simulink model "beta2"  (R2018b)
settings: Solver=FixedStepDiscrete  StartTime=0.0  StopTime=inf  FixedStep=.001  RelTol=1e-3
StartFcn:
  | system('iRobotisManipulator.exe RobotisManipulator_ctr &')
libraries: LibrarySimulinkSAS x4, aerolibanimutils x1
settings Model: SimulationMode=accelerator  Creator=dds  LastModifiedBy=dds
settings OptimizationCC: LifeSpan=inf
settings DebuggingCC: LibraryContextMissingDiagnostic=none  SFExecutionAtInitializationDiag=none
settings SFSimCC: SimUseLocalCustomCode=off
settings RTWCC: RTWUseLocalCustomCode=off
settings CodeAppCC: StateflowObjectComments=on

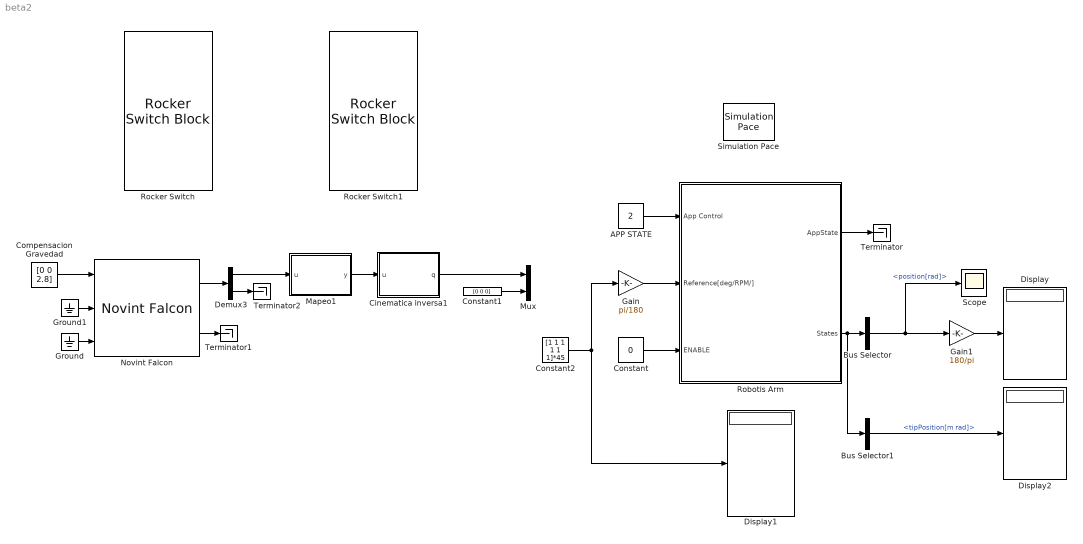
== system beta2 ==
  APP STATE : Constant  Value=2
  Bus Selector : BusSelector  OutputSignals=position[rad]
  Bus Selector1 : BusSelector  OutputSignals=tipPosition[m rad]
  Cinematica inversa1 : MATLAB Function  TreatAsAtomicUnit=on
  Compensacion Gravedad : Constant  Value=[0 0 2.8]  SampleTime=-1
  Constant : Constant  Value=0
  Constant1 : Constant  Value=[0 0 0]
  Constant2 : Constant  Value=[1 1 1 1 1 1]*45
  Demux3 : Demux  Outputs=2
  Display : Display
  Display1 : Display
  Display2 : Display
  Gain : Gain  Gain=pi/180
  Gain1 : Gain  Gain=180/pi
  Ground : Ground
  Ground1 : Ground
  Mapeo1 : MATLAB Function  TreatAsAtomicUnit=on
  Mux : Mux  Inputs=2
  Novint Falcon : LibrarySimulinkSAS/Novint Falcon  dev=1
      settings: SourceProductName=Library SAS
  Robotis Arm : Subsystem  mask{port='COM3', baud='3000000', tloop=10000, ctrType='CTR_POSITION'}
      mask prompts: baud "Baudrate"; tloop "Sample Time [us]"; ctrType "Control Type"
      mask Display:
      | image('robotis.jpg')
      | color('red');
      | port_label('output', 1, 'App ctr State' )
      | port_label('output', 2, 'Robot States' )
      | color('blue');
      | port_label('input', 1, 'App Control')
      | port_label('input', 2, 'Reference [rad]')
      | port_label('input', 3, 'Enable')
      | port_label('input', 4, 'Planes Restriction')
  Rocker Switch : RockerSwitchBlock  WebBlockId=161
      settings: Values={{'CLOSE', 'START'}, [5 2]}
  Rocker Switch1 : RockerSwitchBlock  WebBlockId=162
      settings: Values={{'Motors OFF', 'Motors ON'}, [0 1]}
  Scope : Scope
  Simulation Pace : aerolibanimutils/Simulation Pace  SimulationPace=1  SleepMode=MATLAB Thread  OutputPaceError=off  SampleTime=-1
  Terminator : Terminator
  Terminator1 : Terminator
  Terminator2 : Terminator
  wires:
  APP STATE/1 -> Robotis Arm/1(App Control)
  Constant/1 -> Robotis Arm/3(ENABLE)
  Bus Selector/1 -> Scope/1, Gain1/1  "<position[rad]>"
  Robotis Arm/1(AppState) -> Terminator/1
  Robotis Arm/2(States) -> Bus Selector1/1, Bus Selector/1
  Demux3/2 -> Terminator2/1
  Mapeo1/1(y) -> Cinematica inversa1/1(u)
  Demux3/1 -> Mapeo1/1(u)
  Novint Falcon/1 -> Demux3/1
  Compensacion Gravedad/1 -> Novint Falcon/1
  Ground/1 -> Novint Falcon/3
  Ground1/1 -> Novint Falcon/2
  Novint Falcon/2 -> Terminator1/1
  Cinematica inversa1/1(q) -> Mux/1
  Constant1/1 -> Mux/2
  Gain/1 -> Robotis Arm/2(Reference[deg/RPM/])
  Gain1/1 -> Display/1
  Bus Selector1/1 -> Display2/1  "<tipPosition[m rad]>"
  Constant2/1 -> Gain/1, Display1/1

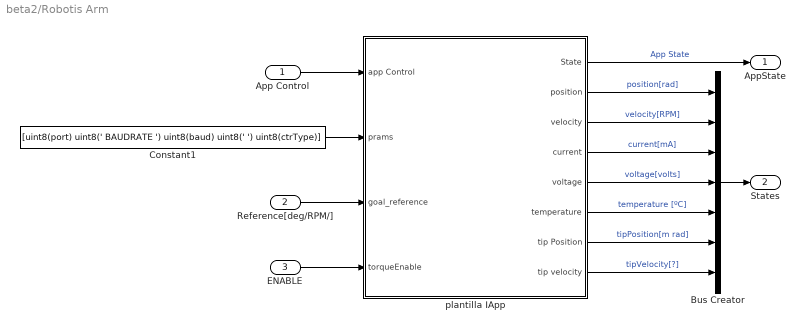
== system beta2/Robotis Arm ==
  App Control : Inport
  Reference[deg/RPM/] : Inport  Port=2
  ENABLE : Inport  Port=3
  Bus Creator : BusCreator  Inputs=7
  Constant1 : Constant  Value=[uint8(port) uint8(' BAUDRATE ') uint8(baud) uint8(' ') uint8(ctrType)]
  plantilla IApp : Subsystem  mask{sys='IServer', shmControl='RobotisManipulator_ctr', shmInput='RobotisManipulator_In', shmOutput='RobotisManipulator_Out', shmInputVect=[6 1], shmOutputVect=[6 6 6 6 6 6 6], shmInputType=['d' 'i'], shmOutputType=['d' 'd' 'd' 'd' 'd' 'd' 'd' ], period=tloop, shmInputOffset=0, shmOutputOffset=0}
      mask prompts: sys "Program"; shmControl "Control Name"; shmInput "Input Name"; shmOutput "OutputName"; shmInputVect "Input Vector"; shmOutputVect "Output Vector"; shmInputType "Input Type"; shmOutputType "Output Type"; period "Period [us]"; shmInputOffset "Input Memory Map Offset"; shmOutputOffset "Output Memory Map Offset"
      mask Display:
      | image('app.png')
      | color('blue');
      | port_label('input', 1, 'App Control')
      | port_label('input', 2, 'prams[char*]')
      | port_label('input', 3, 'goal_reference')
      | port_label('input', 4, 'torqueEnable')
      | color('red');
      | port_label('output', 1, 'App ctr State')
      | port_label('output', 2, 'position')
      | port_label('output', 3, 'velocity')
      | port_label('output', 4, 'current')
      | port_label('output', 5, 'voltage')
      | port_label('output', 6, 'temperature')
      | port_label('output', 7, 'tip position')
      | port_label('output', 8, 'tip velocity')
  AppState : Outport
  States : Outport  Port=2
  wires:
  Reference[deg/RPM/]/1 -> plantilla IApp/3(goal_reference)
  App Control/1 -> plantilla IApp/1(app Control)
  ENABLE/1 -> plantilla IApp/4(torqueEnable)
  plantilla IApp/6(temperature) -> Bus Creator/5  "temperature [ºC]"
  plantilla IApp/1(State) -> AppState/1  "App State"
  plantilla IApp/2(position) -> Bus Creator/1  "position[rad]"
  Bus Creator/1 -> States/1
  Constant1/1 -> plantilla IApp/2(prams)
  plantilla IApp/5(voltage) -> Bus Creator/4  "voltage[volts]"
  plantilla IApp/3(velocity) -> Bus Creator/2  "velocity[RPM]"
  plantilla IApp/4(current) -> Bus Creator/3  "current[mA]"
  plantilla IApp/8(tip velocity) -> Bus Creator/7  "tipVelocity[?]"
  plantilla IApp/7(tip Position) -> Bus Creator/6  "tipPosition[m rad]"

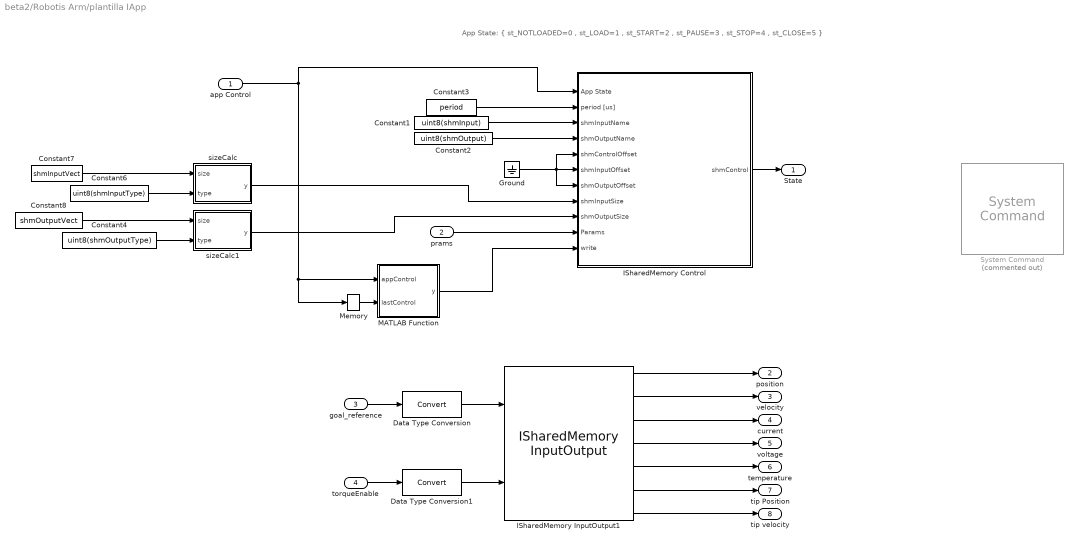
== system beta2/Robotis Arm/plantilla IApp ==
  note: App State: { st_NOTLOADED=0 , st_LOAD=1 , st_START=2 , st_PAUSE=3 , st_STOP=4 , st_CLOSE=5 }
  app Control : Inport
  prams : Inport  Port=2
  goal_reference : Inport  Port=3
  torqueEnable : Inport  Port=4
  Constant1 : Constant  Value=uint8(shmInput)
  Constant2 : Constant  Value=uint8(shmOutput)
  Constant3 : Constant  Value=period
  Constant4 : Constant  Value=uint8(shmOutputType)  OutDataTypeStr=uint8
  Constant6 : Constant  Value=uint8(shmInputType)  OutDataTypeStr=uint8
  Constant7 : Constant  Value=shmInputVect
  Constant8 : Constant  Value=shmOutputVect
  Data Type Conversion : DataTypeConversion
  Data Type Conversion1 : DataTypeConversion
  Ground : Ground
  ISharedMemory Control : Subsystem  AncestorBlock=LibrarySimulinkSAS/ISharedMemory Control  mask{shmControl=shmControl}
      mask prompts: shmControl "Control Name"
      mask Display:
      | image('mem4.png')
      | color('blue');
      | port_label('input', 1, 'App Control')
      | port_label('input', 2, 'Period[us]')
      | port_label('input', 3, 'Input Name')
      | port_label('input', 4, 'Output Name')
      | port_label('input', 5,'Control memory offset')
      | port_label('input', 6,'Input memory offset')
      | port_label('input', 7,'Output memory offset')
      | port_label('input', 8, 'Input Size')
      | port_label('input', 9, 'Output Size')
      | port_label('input', 10, 'Prams')
      | port_label('input', 11, 'Write to mem')
      | color('red');
      | port_label('output', 1, 'App ctr State')
      | port_label('output', 2, 'Error')
  ISharedMemory InputOutput1 : LibrarySimulinkSAS/ISharedMemory InputOutput  nameIn=shmInput  nameOut=shmOutput  vecE=shmInputVect  vecS=shmOutputVect  tipoE=shmInputType  tipoS=shmOutputType  inOff=shmInputOffset  outOff=shmOutputOffset  ts=-1  trigg=off
      settings: SourceProductName=Library SAS
  MATLAB Function : MATLAB Function  TreatAsAtomicUnit=on
  Memory : Memory  InitialCondition=25
  System Command : LibrarySimulinkSAS/System Command  Priority=0  Commented=on  start=' start SASDelay shmcontrol & timeout /t 10'  update=''  outputs=''  terminate='taskkill /IM SASDelay.exe'
      settings: SourceProductName=Library SAS
  sizeCalc : MATLAB Function  TreatAsAtomicUnit=on
  sizeCalc1 : MATLAB Function  TreatAsAtomicUnit=on
  State : Outport
  position : Outport  Port=2
  velocity : Outport  Port=3
  current : Outport  Port=4
  voltage : Outport  Port=5
  temperature : Outport  Port=6
  tip Position : Outport  Port=7
  tip velocity : Outport  Port=8
  wires:
  Ground/1 -> ISharedMemory Control/6(shmInputOffset), ISharedMemory Control/5(shmControlOffset), ISharedMemory Control/7(shmOutputOffset)
  goal_reference/1 -> Data Type Conversion/1
  Constant4/1 -> sizeCalc1/2(type)
  Constant8/1 -> sizeCalc1/1(size)
  Constant6/1 -> sizeCalc/2(type)
  Constant7/1 -> sizeCalc/1(size)
  sizeCalc/1(y) -> ISharedMemory Control/8(shmInputSize)
  prams/1 -> ISharedMemory Control/10(Params)
  sizeCalc1/1(y) -> ISharedMemory Control/9(shmOutputSize)
  Memory/1 -> MATLAB Function/2(lastControl)
  Constant3/1 -> ISharedMemory Control/2(period [us])
  app Control/1 -> MATLAB Function/1(appControl), Memory/1, ISharedMemory Control/1(App State)
  ISharedMemory Control/1(shmControl) -> State/1
  Constant1/1 -> ISharedMemory Control/3(shmInputName)
  Constant2/1 -> ISharedMemory Control/4(shmOutputName)
  MATLAB Function/1(y) -> ISharedMemory Control/11(write)
  torqueEnable/1 -> Data Type Conversion1/1
  Data Type Conversion/1 -> ISharedMemory InputOutput1/1
  Data Type Conversion1/1 -> ISharedMemory InputOutput1/2
  ISharedMemory InputOutput1/1 -> position/1
  ISharedMemory InputOutput1/2 -> velocity/1
  ISharedMemory InputOutput1/3 -> current/1
  ISharedMemory InputOutput1/4 -> voltage/1
  ISharedMemory InputOutput1/5 -> temperature/1
  ISharedMemory InputOutput1/7 -> tip velocity/1
  ISharedMemory InputOutput1/6 -> tip Position/1

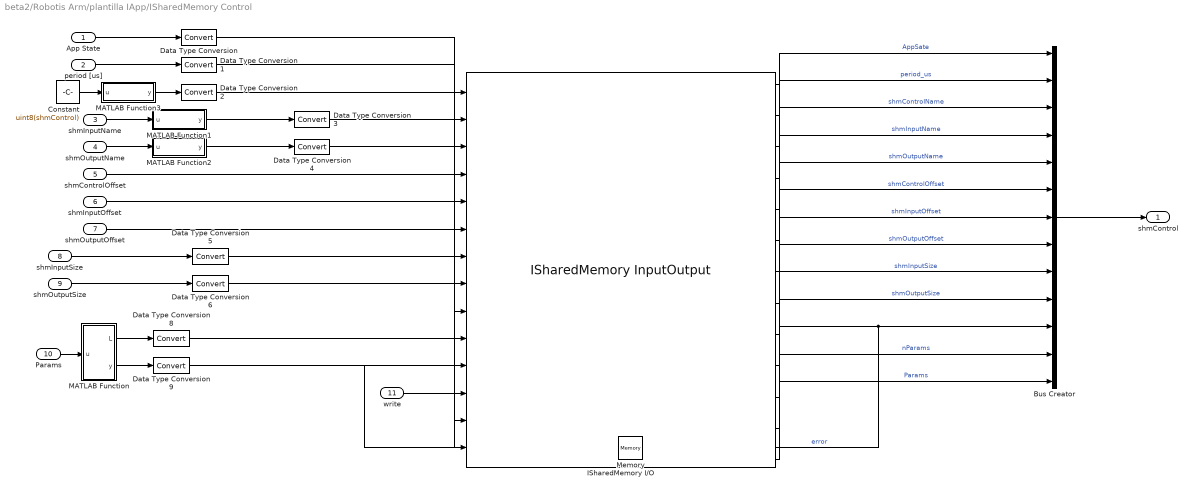
== system beta2/Robotis Arm/plantilla IApp/ISharedMemory Control ==
  App State : Inport
  period [us] : Inport  Port=2
  shmInputName : Inport  Port=3
  shmOutputName : Inport  Port=4
  shmControlOffset : Inport  Port=5
  shmInputOffset : Inport  Port=6
  shmOutputOffset : Inport  Port=7
  shmInputSize : Inport  Port=8
  shmOutputSize : Inport  Port=9
  Params : Inport  Port=10
  write : Inport  Port=11
  Bus Creator : BusCreator  Inputs=13
  Constant : Constant  Value=uint8(shmControl)
  Data Type Conversion{,1..6,8..9} (9 alike) : DataTypeConversion
  ISharedMemory I/O : LibrarySimulinkSAS/ISharedMemory InputOutput  Priority=10  nameIn=shmControl  nameOut=shmControl  vecE=[1 1 40 40 40 1 1 1 1 1 1 1 400]  vecS=[1 1 40 40 40 1 1 1 1 1 1 1 400]  tipoE=['i' 'i' 'c' 'c' 'c' 'i' 'i' 'i' 'i' 'i' 'i' 'i' 'c']  tipoS=['i' 'i' 'c' 'c' 'c' 'i' 'i' 'i' 'i' 'i' 'i' 'i' 'c']  inOff=0  outOff=0  ts=-1  trigg=on
      settings: SourceProductName=Library SAS
  MATLAB Function : MATLAB Function  TreatAsAtomicUnit=on
  MATLAB Function1 : MATLAB Function  TreatAsAtomicUnit=on
  MATLAB Function2 : MATLAB Function  TreatAsAtomicUnit=on
  MATLAB Function3 : MATLAB Function  TreatAsAtomicUnit=on
  Memory : Memory
  shmControl : Outport
  wires:
  ISharedMemory I/O/2 -> Bus Creator/2  "period_us"
  ISharedMemory I/O/3 -> Bus Creator/3  "shmControlName"
  Memory/1 -> ISharedMemory I/O/11
  ISharedMemory I/O/1 -> Bus Creator/1  "AppSate"
  MATLAB Function/1(L) -> Data Type Conversion8/1
  MATLAB Function3/1(y) -> Data Type Conversion2/1
  MATLAB Function2/1(y) -> Data Type Conversion4/1
  MATLAB Function1/1(y) -> Data Type Conversion3/1
  MATLAB Function/2(y) -> Data Type Conversion9/1
  shmInputName/1 -> MATLAB Function1/1(u)
  shmInputSize/1 -> Data Type Conversion5/1
  shmOutputName/1 -> MATLAB Function2/1(u)
  shmOutputSize/1 -> Data Type Conversion6/1
  Params/1 -> MATLAB Function/1(u)
  App State/1 -> Data Type Conversion/1
  period [us]/1 -> Data Type Conversion1/1
  write/1 -> ISharedMemory I/O/14
  Data Type Conversion9/1 -> ISharedMemory I/O/13
  Data Type Conversion8/1 -> ISharedMemory I/O/12
  ISharedMemory I/O/11 -> Bus Creator/11, Memory/1  "error"
  Data Type Conversion6/1 -> ISharedMemory I/O/10
  Data Type Conversion5/1 -> ISharedMemory I/O/9
  Data Type Conversion/1 -> ISharedMemory I/O/1
  Data Type Conversion1/1 -> ISharedMemory I/O/2
  Data Type Conversion2/1 -> ISharedMemory I/O/3
  Data Type Conversion4/1 -> ISharedMemory I/O/5
  Data Type Conversion3/1 -> ISharedMemory I/O/4
  shmControlOffset/1 -> ISharedMemory I/O/6
  shmInputOffset/1 -> ISharedMemory I/O/7
  shmOutputOffset/1 -> ISharedMemory I/O/8
  Constant/1 -> MATLAB Function3/1(u)
  ISharedMemory I/O/4 -> Bus Creator/4  "shmInputName"
  ISharedMemory I/O/5 -> Bus Creator/5  "shmOutputName"
  ISharedMemory I/O/6 -> Bus Creator/6  "shmControlOffset"
  ISharedMemory I/O/7 -> Bus Creator/7  "shmInputOffset"
  ISharedMemory I/O/8 -> Bus Creator/8  "shmOutputOffset"
  ISharedMemory I/O/9 -> Bus Creator/9  "shmInputSize"
  ISharedMemory I/O/10 -> Bus Creator/10  "shmOutputSize"
  ISharedMemory I/O/12 -> Bus Creator/12  "nParams"
  ISharedMemory I/O/13 -> Bus Creator/13  "Params"
  Bus Creator/1 -> shmControl/1

== matlab function beta2/Robotis Arm/plantilla IApp/MATLAB Function ==
  data: appControl input; lastControl input; y output
function y = fcn(appControl,lastControl)
if(appControl~=lastControl)
    y=1;
else
    y=0;
end

== matlab function beta2/Robotis Arm/plantilla IApp/ISharedMemory Control/MATLAB Function3 ==
  data: u input; y output
function y = fcn(u)
y=zeros(40,1);
y(1:length(u),1)=u;

== matlab function beta2/Robotis Arm/plantilla IApp/sizeCalc ==
  data: size input; y output; type input
function y = fcn(size,type)
n=length(size);
y=0;
for i=1:n
    switch type(i)
        case 'c'
            aux=size(i)*1;
        case 'C'
            aux=size(i)*1;
        case 'd'
            aux=size(i)*6;
        case 'f'
            aux=size(i)*4;
        case 'i'
            aux=size(i)*4;
        case 'I'
            aux=size(i)*4;
        otherwise %double
            aux=size(i)*6;
    end
y=y+aux;
end
end

== matlab function beta2/Robotis Arm/plantilla IApp/ISharedMemory Control/MATLAB Function ==
  data: L output; u input; y output
function [L,y] = fcn(u)
y=zeros(400,1);
L=length(u);
y(1:L,1)=u;

== matlab function beta2/Robotis Arm/plantilla IApp/ISharedMemory Control/MATLAB Function1 ==
  data: u input; y output
function y = fcn(u)
y=zeros(40,1);
y(1:length(u),1)=u;

== matlab function beta2/Robotis Arm/plantilla IApp/ISharedMemory Control/MATLAB Function2 ==
  data: u input; y output
function y = fcn(u)
y=zeros(40,1);
y(1:length(u),1)=u;

== matlab function beta2/Robotis Arm/plantilla IApp/sizeCalc1 ==
  data: size input; y output; type input
function y = fcn(size,type)
n=length(size);
y=0;
for i=1:n
    switch type(i)
        case 'c'
            aux=size(i)*1;
        case 'C'
            aux=size(i)*1;
        case 'd'
            aux=size(i)*6;
        case 'f'
            aux=size(i)*4;
        case 'i'
            aux=size(i)*4;
        case 'I'
            aux=size(i)*4;
        otherwise %double
            aux=size(i)*6;
    end
y=y+aux;
end
end

== matlab function beta2/Cinematica inversa1 ==
  data: u input; q output
function q  = fcn(u)
%#codegen

x=u(1);
y=u(2);
z=u(3);

if(x<5)
    x=5;
end

if(z<25)
    z=25;
end


AltoTorso=30.0;
AnchoTorso=30;
L1=15.9;
L2=26.4;
L3=25.8;
L4=12.3;



%r.teach([0 0 0 0 0])


deltaX=x;
deltaY=y;
deltaZ=z;


q1=(180/pi)*atan2(deltaY,deltaX);

if(q1>180)
    q1=q1-360;
end

if(q1<-180)
    q1=q1+360;
end

if(q1>180)
    q1=180;
end

if(q1<-180)
    q1=-180;
end

aux=(deltaX^2+deltaY^2+(deltaZ-L1)^2-L2^2-L3^2)/(2*L2*L3);

if(aux>1)
    aux=1;
end

if(aux<-1)
    aux=-1;
end


q3=acos(aux);


q2=atan2(sqrt(deltaX^2+deltaY^2),deltaZ-L1)-atan2(L3*sin(q3),L2+L3*cos(q3));
q2=(180/pi)*q2;

if(q2>90)
    q2=90;
end

if(q2<-90)
    q2=-90;
end


q3=(180/pi)*q3;

if(q3>135)
    q3=135;
end

if(q3<-90)
    q3=-90;
end

q=[q1;q2;q3-45];

== matlab function beta2/Mapeo1 ==
  data: u input; y output
function y = fcn(u)
%#codegen

Xnovint=u(1);
Ynovint=u(2);
Znovint=u(3);

Xlim=5;
Ylim=5.5;
Zlim=[-4.5 2.5];

if(Xnovint>Xlim)
    Xnovint=Xlim;
end

if(Xnovint<-Xlim)
    Xnovint=-Xlim;
end

if(Ynovint>Ylim)
    Ynovint=Ylim;
end

if(Ynovint<-Ylim)
    Ynovint=-Ylim;
end

if(Znovint<Zlim(1))
    Znovint=Zlim(1);
end

if(Znovint>Zlim(2))
    Znovint=Zlim(2);
end


Yrobot=(40/5)*Xnovint;

Xrobot=(50/(2*5.5))*(Ynovint+5.5);

Zrobot=(50/7)*(Znovint+4.5)+25;

y=u;

y(1) = Xrobot;
y(2) = -Yrobot;
y(3) = Zrobot;
